simulink model "CSAD_model"  (R2016b)
settings: Solver=ode5  StartTime=0.0  StopTime=t_sim  FixedStep=0.01  RelTol=1e-3
undefined symbols (not defined in the file or in its folder): eta_initial, Gamma1, Gamma2, nu_initial
settings Model: Creator=torees  LastModifiedBy=utente

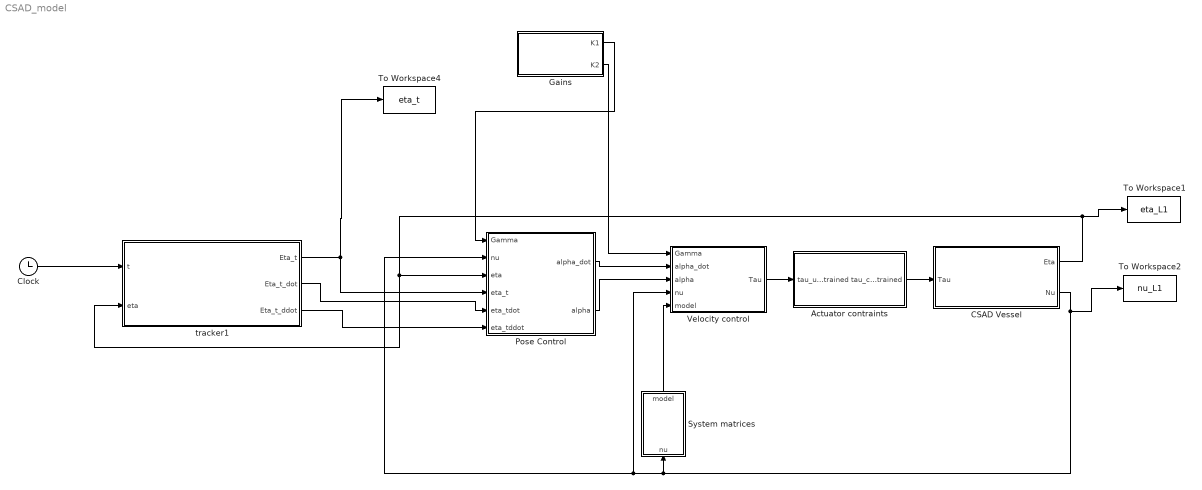
== system CSAD_model ==
  Actuator contraints : Subsystem
  CSAD Vessel : Subsystem
  Clock : Clock
  Gains : Subsystem
  Pose Control : Subsystem
  System matrices : MATLAB Function  TreatAsAtomicUnit=on
  To Workspace1 : ToWorkspace  VariableName=eta_L1  SampleTime=-1
  To Workspace2 : ToWorkspace  VariableName=nu_L1  SampleTime=-1
  To Workspace4 : ToWorkspace  VariableName=eta_t  SampleTime=-1
  Velocity control : Subsystem
  tracker1 : MATLAB Function  TreatAsAtomicUnit=on
  wires:
  Clock/1 -> tracker1/1(t)
  tracker1/1(Eta_t) -> To Workspace4/1, Pose Control/4(eta_t)
  Pose Control/2(alpha) -> Velocity control/3(alpha)
  Pose Control/1(alpha_dot) -> Velocity control/2(alpha_dot)
  System matrices/1(model) -> Velocity control/5(model)
  CSAD Vessel/2(Nu) -> To Workspace2/1, System matrices/1(nu), Velocity control/4(nu), Pose Control/2(nu)
  tracker1/2(Eta_t_dot) -> Pose Control/5(eta_tdot)
  tracker1/3(Eta_t_ddot) -> Pose Control/6(eta_tddot)
  CSAD Vessel/1(Eta) -> To Workspace1/1, Pose Control/3(eta), tracker1/2(eta)
  Gains/1(K1) -> Pose Control/1(Gamma)
  Gains/2(K2) -> Velocity control/1(Gamma)
  Velocity control/1(Tau) -> Actuator contraints/1(tau_unconstrained)
  Actuator contraints/1(tau_contrained) -> CSAD Vessel/1(Tau)

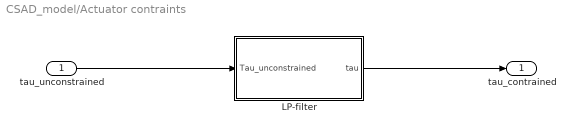
== system CSAD_model/Actuator contraints ==
  tau_unconstrained : Inport
  LP-filter : Subsystem
  tau_contrained : Outport
  wires:
  LP-filter/1(tau) -> tau_contrained/1
  tau_unconstrained/1 -> LP-filter/1(Tau_unconstrained)

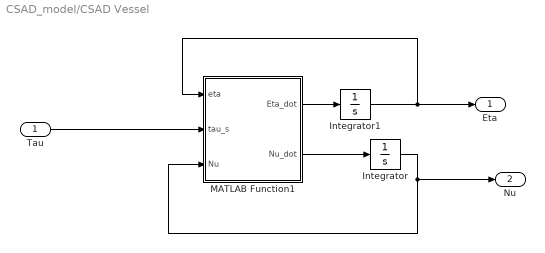
== system CSAD_model/CSAD Vessel ==
  Tau : Inport
  Integrator : Integrator  InitialCondition=nu_initial
  Integrator1 : Integrator  InitialCondition=eta_initial
  MATLAB Function1 : MATLAB Function  TreatAsAtomicUnit=on
  Eta : Outport
  Nu : Outport  Port=2
  wires:
  Integrator/1 -> Nu/1, MATLAB Function1/3(Nu)
  MATLAB Function1/1(Eta_dot) -> Integrator1/1
  Integrator1/1 -> Eta/1, MATLAB Function1/1(eta)
  MATLAB Function1/2(Nu_dot) -> Integrator/1
  Tau/1 -> MATLAB Function1/2(tau_s)

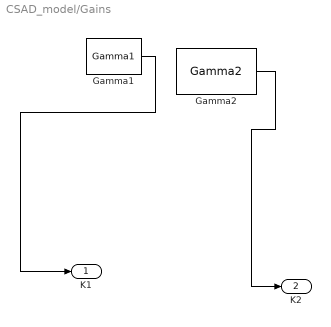
== system CSAD_model/Gains ==
  Gamma1 : Constant  Value=Gamma1
  Gamma2 : Constant  Value=Gamma2
  K1 : Outport
  K2 : Outport  Port=2
  wires:
  Gamma2/1 -> K2/1
  Gamma1/1 -> K1/1

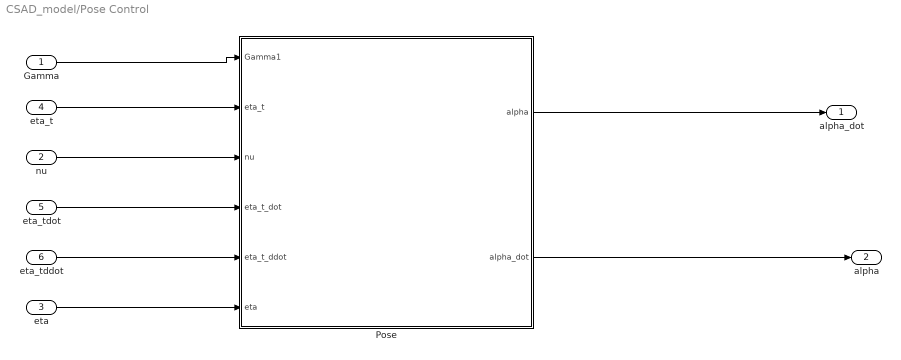
== system CSAD_model/Pose Control ==
  Gamma : Inport
  nu : Inport  Port=2
  eta : Inport  Port=3
  eta_t : Inport  Port=4
  eta_tdot : Inport  Port=5
  eta_tddot : Inport  Port=6
  Pose : MATLAB Function  TreatAsAtomicUnit=on
  alpha_dot : Outport
  alpha : Outport  Port=2
  wires:
  Pose/1(alpha) -> alpha_dot/1
  Pose/2(alpha_dot) -> alpha/1
  eta/1 -> Pose/6(eta)
  eta_tdot/1 -> Pose/4(eta_t_dot)
  eta_tddot/1 -> Pose/5(eta_t_ddot)
  eta_t/1 -> Pose/2(eta_t)
  nu/1 -> Pose/3(nu)
  Gamma/1 -> Pose/1(Gamma1)

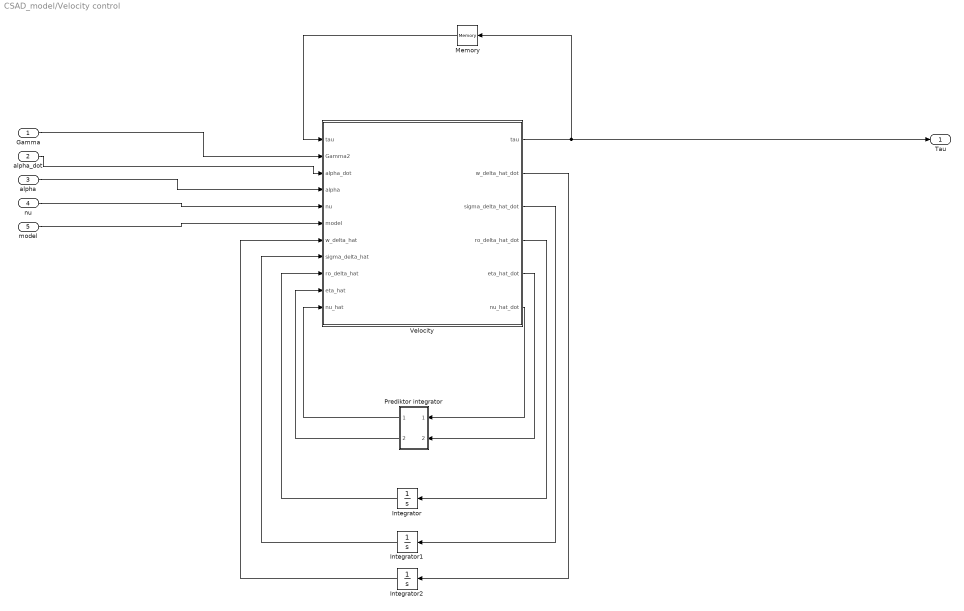
== system CSAD_model/Velocity control ==
  Gamma : Inport
  alpha_dot : Inport  Port=2
  alpha : Inport  Port=3
  nu : Inport  Port=4
  model : Inport  Port=5
  Integrator : Integrator  InitialCondition=1
  Integrator1 : Integrator  InitialCondition=1
  Integrator2 : Integrator  InitialCondition=[0, 0, 0]'
  Memory : Memory  X0=[0 0 0]
  Prediktor integrator : Subsystem
  Velocity : MATLAB Function  TreatAsAtomicUnit=on
  Tau : Outport
  wires:
  alpha_dot/1 -> Velocity/3(alpha_dot)
  alpha/1 -> Velocity/4(alpha)
  nu/1 -> Velocity/5(nu)
  model/1 -> Velocity/6(model)
  Gamma/1 -> Velocity/2(Gamma2)
  Prediktor integrator/1(Out2) -> Velocity/11(nu_hat)
  Velocity/3(sigma_delta_hat_dot) -> Integrator1/1
  Velocity/6(nu_hat_dot) -> Prediktor integrator/1(In2)
  Integrator1/1 -> Velocity/8(sigma_delta_hat)
  Velocity/5(eta_hat_dot) -> Prediktor integrator/2(In1)
  Velocity/4(ro_delta_hat_dot) -> Integrator/1
  Integrator2/1 -> Velocity/7(w_delta_hat)
  Prediktor integrator/2(Out1) -> Velocity/10(eta_hat)
  Velocity/2(w_delta_hat_dot) -> Integrator2/1
  Integrator/1 -> Velocity/9(ro_delta_hat)
  Memory/1 -> Velocity/1("tau ")
  Velocity/1(tau) -> Tau/1, Memory/1

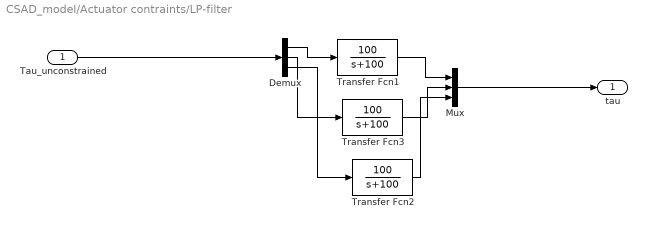
== system CSAD_model/Actuator contraints/LP-filter ==
  Tau_unconstrained : Inport
  Demux : Demux  Outputs=3
  Mux : Mux  Inputs=3
  Transfer Fcn1 : TransferFcn  Numerator=[100]  Denominator=[1 100]
  Transfer Fcn2 : TransferFcn  Numerator=[100]  Denominator=[1 100]
  Transfer Fcn3 : TransferFcn  Numerator=[100]  Denominator=[1 100]
  tau : Outport
  wires:
  Transfer Fcn1/1 -> Mux/1
  Demux/2 -> Transfer Fcn3/1
  Mux/1 -> tau/1
  Demux/1 -> Transfer Fcn1/1
  Transfer Fcn2/1 -> Mux/3
  Transfer Fcn3/1 -> Mux/2
  Demux/3 -> Transfer Fcn2/1
  Tau_unconstrained/1 -> Demux/1

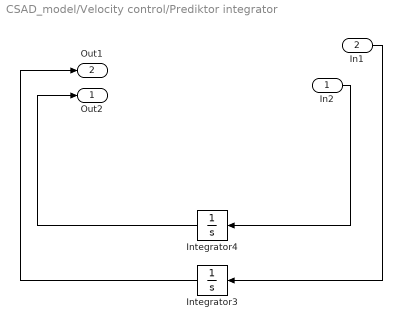
== system CSAD_model/Velocity control/Prediktor integrator ==
  In2 : Inport
  In1 : Inport  Port=2
  Integrator3 : Integrator  InitialCondition=eta_initial
  Integrator4 : Integrator  InitialCondition=nu_initial
  Out2 : Outport
  Out1 : Outport  Port=2
  wires:
  Integrator3/1 -> Out1/1
  Integrator4/1 -> Out2/1
  In1/1 -> Integrator3/1
  In2/1 -> Integrator4/1

== matlab function CSAD_model/Pose Control/Pose ==
  data: Gamma1 input; eta_t input; nu input; eta_t_dot input; eta_t_ddot input; alpha output; alpha_dot output; eta input
function [alpha,alpha_dot]= fcn(Gamma1,eta_t,nu,eta_t_dot,eta_t_ddot,eta)

psi=eta(3);
r=nu(3);
R_T = [cos(psi) -sin(psi) 0;
       sin(psi) cos(psi) 0;
       0 0 1]';
S_T = [0 -r 0;
        r 0 0;
        0 0 0]';

z_1 = R_T*(eta-eta_t);

z1_p_tilde = [z_1(1) z_1(2)]';
z1_psi_tilde = z_1(3);
delta_p_tilde = 0.4;
delta_psi_tilde = 0.4;


K1_func = Gamma1*[ 1/sqrt(z1_p_tilde'*z1_p_tilde + delta_p_tilde^2) 0 0;
                0 1/sqrt(z1_p_tilde'*z1_p_tilde + delta_p_tilde^2) 0;
                0 0 1/sqrt(z1_psi_tilde^2 + delta_psi_tilde^2)];

alpha = R_T*eta_t_dot - K1_func*z_1;            
z_2 = nu-alpha;
z_1_dot = S_T*z_1 - Gamma1*z_1 + z_2;
z1_p_tilde_dot = [z_1_dot(1) z_1_dot(2)]';
z1_psi_tilde_dot = z_1_dot(3);
K1_func_dot = -Gamma1*[z1_p_tilde'*z1_p_tilde_dot/((z1_p_tilde'*z1_p_tilde+delta_p_tilde^2)^(3/2)) 0 0;
                0 z1_p_tilde'*z1_p_tilde_dot/((z1_p_tilde'*z1_p_tilde+delta_p_tilde^2)^(3/2)) 0;
                0 0 z1_psi_tilde*z1_psi_tilde_dot/((z1_psi_tilde^2+delta_psi_tilde^2)^(3/2))];

alpha_dot = R_T*eta_t_ddot + S_T*R_T*eta_tdot - K1_func_dot*z_1 - K1_func*z_1_dot;

== matlab function CSAD_model/Velocity control/Velocity ==
  data: tau input; Gamma2 input; alpha_dot input; alpha input; tau output; nu input; model input; w_delta_hat input; sigma_delta_hat input; ro_delta_hat input; eta_hat input; nu_hat input; w_delta_hat_dot output; sigma_delta_hat_dot output; ro_delta_hat_dot output; eta_hat_dot output; nu_hat_dot output
function [tau,w_delta_hat_dot,sigma_delta_hat_dot,ro_delta_hat_dot,eta_hat_dot,nu_hat_dot]= fcn(tau,Gamma2,alpha_dot,alpha,nu,model,w_delta_hat,sigma_delta_hat,ro_delta_hat,eta_hat,nu_hat)
z2=nu-alpha;

M = model(1:3,1:3);
C = model(1:3,4:6);
D = model(1:3,7:9);
psi=eta(3);
R_T = [cos(psi) -sin(psi) 0;
       sin(psi) cos(psi) 0;
       0 0 1]';
eta_tilde = eta_hat - eta;
nu_tilde = nu_hat - nu;

z2_nu_tilde = [z2(1) z2(2)]';
z2_r_tilde = z2(3);

delta_nu_tilde = 0.8;
delta_r_tilde = 0.02;

K2_func = Gamma2*[ 1/sqrt(z2_nu_tilde'*z2_nu_tilde+delta_nu_tilde^2) 0 0;
    0 1/sqrt(z2_nu_tilde'*z2_nu_tilde+delta_nu_tilde^2) 0;
    0 0 1/sqrt(z2_r_tilde^2+delta_r_tilde^2)];


%adapt gains
K1 =diag([0.05,0.05,0.02]*10);
K2 =diag([5,7,15]*2);
gamma_ro_delta=100;
gamma_sigma_delta=100;
gamma_w_delta = 30; 
L1 = eye(3)*2*K1;
L2 = eye(3)*2*K2;



%%adaptation laws
ro_delta_hat_dot = -gamma_ro_delta*nu_tilde'*tau;
sigma_delta_hat_dot = gamma_sigma_delta*nu_tilde'*D*nu;
w_delta_hat_dot=-gamma_w_delta*R_T'*nu_tilde;

%%State predictor dynamics
eta_hat_dot = -L1*eta_tilde + R_T'*nu;
nu_hat_dot = -L2*nu_tilde + M\(ro_delta_hat*tau+R_T*w_delta_hat-C*nu-sigma_delta_hat*D*nu);

tau =(-R_T*w_delta_hat + M*alpha_dot + C*nu + sigma_delta_hat*D*nu - K2_func*z2)/ro_delta_hat;

== matlab function CSAD_model/System matrices ==
  data: model output; nu input
function model = fcn(nu)

X_u		= -2.332;		
X_uu 	=  0;		
X_uuu	= -8.557;

Y_v		= -4.673;   
Y_vv	= - 0.3976;
Y_vvv	= -313.3;	
Y_r		= -7.25;
Y_rr	= -3.45;
Y_rrr   = 0;

N_v		= 0;		
N_vv	= -0.2088;
N_vvv = 0;

N_r		= -7.141;
N_rr	= -4.888;
N_rrr	= -0.152;

N_rv	= 0.08;	
N_vr	= 0.08;
Y_rv	= -0.805;			
Y_vr	= -0.845;

X_ud =     -3.262;
Y_vd =     -28.89;
Y_rd =     -0.525;
N_vd =     -0.157;	
N_rd =     -13.98;

Nur  = -Y_rd;
Nuv  = -(Y_vd-X_ud);
Yur  = -X_ud;

x_g     = 0.0375;
m       = 127.92;
I_z     = 61.967;

u   = Nu(1);
v   = Nu(2);
r   = Nu(3);

d_11 = - X_u - X_uu*abs(u) - X_uuu*u^2;
d_22 = - Y_v - Y_vv*abs(v) - Y_rv*abs(r) - Y_vvv*v^2;
d_23 = - Y_r - Y_rr*abs(r) - Y_vr*abs(v) - Y_rrr*r^2 - Yur*u;
d_32 = - N_v - N_vv*abs(v) - N_rv*abs(r) - N_vvv*v^2 - Nuv*u;
d_33 = - N_r - N_rr*abs(r) - N_vr*abs(v) - N_rrr*r^2 - Nur*u;

D    = [d_11  0     0
        0     d_22  d_23
        0     d_32  d_33];

CA=[0                            0          Y_vd*v+Y_rd*r;
    0                            0                -X_ud*u;
    -Y_rd*r-Y_vd*v               X_ud*u                0];

CRB=[0             0     -m*(x_g*r+v);
     0             0      m*u;
     m*(x_g*r+v) -m*u     0]; 

C=CRB+CA;

M_RB_c=[m     0      0;
        0     m      m*x_g;
        0     m*x_g  I_z];

M_A_c=[-X_ud    0      0;
         0    -Y_vd  -Y_rd;
         0    -N_vd  -N_rd];     
    
M = M_RB_c + M_A_c;
model=[M C D];

== matlab function CSAD_model/tracker1 ==
  data: t input; Eta_t output; Eta_t_dot output; Eta_t_ddot output; eta input
function [ Eta_t, Eta_t_dot, Eta_t_ddot]   = tracking(t,eta)

v_t = 0.15;

etaP = [5 7 7 7 5 5;
       -1 -1 1 1 1 -1;
        0 0 0 pi/4 pi/4 0];
Eta_t_dot = [0;0;0];
Eta_t_ddot = [0;0;0];

Eta_t = [5;-1;0];
persistent point ;
if(isempty(point))
    point = 1;
    
end



switch point
    case 1
        Eta_t = etaP(:,2);
         if ((abs((Eta_t(1)- eta(1))) <0.01 ) ==1  ) && ((abs(Eta_t(2)-eta(2))<0.01) ==1) && (abs(Eta_t(3)-rad2deg(eta(3)))<1 == 1)
            point = 2;
            return;
         end
        
        
    case 2
        Eta_t = etaP(:,3);
        if((abs((Eta_t(1)- eta(1))) <0.01 ) ==1  ) && ((abs(Eta_t(2)-eta(2))<0.01) ==1) && (abs(Eta_t(3)-rad2deg(eta(3)))<1 == 1) 
            point = 3;
            return;
         end
    case 3
        Eta_t = etaP(:,4);
        if((abs((Eta_t(1)- eta(1))) <0.01 ) ==1  ) && ((abs(Eta_t(2)-eta(2))<0.01) ==1) && (rad2deg(abs(Eta_t(3)-eta(3)))<1 == 1)  
            point = 4;
            return;
            
         end
    case 4
        Eta_t = etaP(:,5);
        if((abs((Eta_t(1)- eta(1))) <0.01 ) ==1  ) && ((abs(Eta_t(2)-eta(2))<0.01) ==1) && (rad2deg(abs(Eta_t(3)-eta(3)))<1 == 1) 
            point = 5; 
            return;
         end
    case 5
        Eta_t = etaP(:,6);
        if((abs((Eta_t(1)- eta(1))) <0.01 ) ==1  ) && ((abs(Eta_t(2)-eta(2))<0.01) ==1) && (abs(Eta_t(3)-rad2deg(eta(3)))<1 == 1) 
            point = 6; 
            return;
         end

    otherwise
        

end
end
%(abs(Eta_t(2)-eta(2))<0.01) &&

== matlab function CSAD_model/CSAD Vessel/MATLAB Function1 ==
  data: eta input; tau_s input; Eta_dot output; Nu input; Nu_dot output
function [Eta_dot,Nu_dot] = Vessel(eta,tau_s,Nu)

Nu_dot = CSAD_full(Nu,tau_s);

yaw = eta(3);

R =[cos(yaw) -sin(yaw) 0;
            sin(yaw)  cos(yaw) 0;
            0         0        1]; 
Eta_dot = R*Nu;
end
